simulink model "Calculator"  (R2021a)
settings: Solver=FixedStepDiscrete  StartTime=0.0  StopTime=10.0  RelTol=1e-3
libraries: simulink x1
settings Model: SimulationMode=accelerator  Creator=hp  LastModifiedBy=hp
settings OptimizationCC: DefaultParameterBehavior=Inlined  EnhancedBackFolding=on  PassReuseOutputArgsAs=Individual arguments  ZeroExternalMemoryAtStartup=off  ZeroInternalMemoryAtStartup=off  OptimizeBlockOrder=speed  DifferentSizesBufferReuse=on  OptimizationCustomize=off  EfficientTunableParamExpr=on
settings DebuggingCC: ParameterTunabilityLossMsg=error
settings SFSimCC: MATLABDynamicMemAlloc=off
settings RTWCC: SystemTargetFile=ert.tlc  GenCodeOnly=on  TemplateMakefile=ert_default_tmf  GenerateReport=on  IncludeHyperlinkInReport=on  LaunchReport=on  GenerateTraceInfo=on
settings CodeAppCC: ForceParamTrailComments=on  IgnoreCustomStorageClasses=off  OperatorAnnotations=on  SimulinkDataObjDesc=on  SFDataObjDesc=on  InsertBlockDesc=on
settings ERTTargetCC: TargetLangStandard=C99 (ISO)  GenerateSampleERTMain=on  SupportNonFinite=off  SupportComplex=off  InlinedParameterPlacement=NonHierarchical  ERTCustomFileTemplate=example_file_process.tlc  IndentSize=4  EnableUserReplacementTypes=on

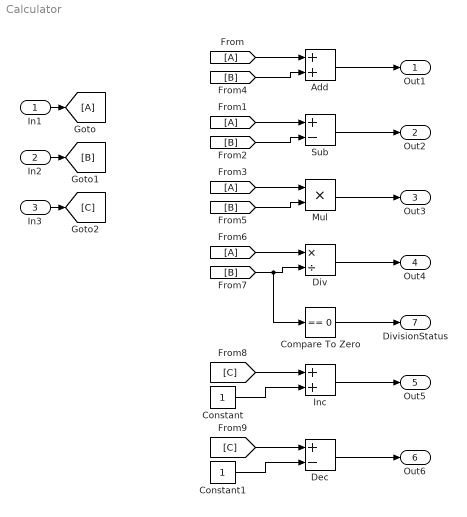
== system Calculator ==
  In1 : Inport  OutDataTypeStr=double
  In2 : Inport  Port=2  OutDataTypeStr=double
  In3 : Inport  Port=3  OutDataTypeStr=double
  Add : Sum
  Compare To Zero : simulink/Logic and Bit Operations/Compare To Zero  relop===  OutDataTypeStr=boolean
  Constant : Constant
  Constant1 : Constant
  Dec : Sum  Inputs=+-
  Div : Product  Inputs=*/
  Inc : Sum
  Mul : Product  Inputs=**
  Sub : Sum  Inputs=+-
  Out1 : Outport
  Out2 : Outport  Port=2
  Out3 : Outport  Port=3
  Out4 : Outport  Port=4
  Out5 : Outport  Port=5
  Out6 : Outport  Port=6
  DivisionStatus : Outport  Port=7
  wires:
  In1/1 -> [A]
  [A] -> Add/1
  In2/1 -> [B]
  [B] -> Add/2
  [B] -> Sub/2
  [A] -> Sub/1
  [B] -> Mul/2
  [A] -> Mul/1
  [B] -> Div/2, Compare To Zero/1
  [A] -> Div/1
  In3/1 -> [C]
  [C] -> Inc/1
  Constant/1 -> Inc/2
  Constant1/1 -> Dec/2
  [C] -> Dec/1
  Add/1 -> Out1/1
  Sub/1 -> Out2/1
  Mul/1 -> Out3/1
  Div/1 -> Out4/1
  Inc/1 -> Out5/1
  Dec/1 -> Out6/1
  Compare To Zero/1 -> DivisionStatus/1
